simulink model "Encoder_polling"  (R2024b)
settings: Solver=FixedStepAuto  StartTime=0.0  StopTime=inf  FixedStep=0.001  RelTol=1e-3  EnableMultiTasking=on
libraries: stm32f4xxblockslib x5, stm32g4xxblockslib x3, simulink_extras x1
settings Model: STM32="{\"DigitalPortRead\":[{\"ID\":\"untitled:9\"},{\"ID\":\"untitled:10\"},{\"ID\":\"Encoder_Sim:129\"},{\"ID\":\"Encoder_Sim:130\"},{\"ID\":\"Encoder_Sim:134\"},{\"ID\":\"Encoder_Sim:135\"},{\"ID\":\"Encoder_Sim:299\"},{\"ID\":\"Encoder_polling:299\"},{\"ID\":\"Encoder_polling:130\"},{\"ID\":\"Encoder_polling:129\"},{\"ID\":\"Encoder_polling:135\"},{\"ID\":\"Encoder_polling:134\"}],\"EncoderBlockForG4\":[{\"ID\":\"untitled:13\"},{\"ID\":\"untitled:14\"},{\"ID\":\"untitled:15\"},{\"ID\":\"Encoder_Sim:13\"},{\"ID\":\"Encoder_Sim:14\"},{\"ID\":\"Encoder_Sim:15\"}]}"  Creator=chant  LastModifiedBy=pongn
settings OptimizationCC: BlockReduction=off  BooleanDataType=off  DefaultParameterBehavior=Inlined  EnhancedBackFolding=on  PassReuseOutputArgsAs=Individual arguments  ZeroExternalMemoryAtStartup=off  ZeroInternalMemoryAtStartup=off  MaxStackSize=512  OptimizeBlockOrder=speed  DifferentSizesBufferReuse=on  OptimizationCustomize=off  EfficientTunableParamExpr=on
settings DebuggingCC: SaveWithParameterizedLinksMsg=none  UnderspecifiedInitializationDetection=Classic  MergeDetectMultiDrivingBlocksExec=none  SignalResolutionControl=TryResolveAllWithWarning  ParameterTunabilityLossMsg=error
settings HardwareCC: ProdBitPerPointer=32  ProdBitPerSizeT=32  ProdBitPerPtrDiffT=32  ProdLargestAtomicInteger=Long  ProdLargestAtomicFloat=Double  ProdWordSize=32  ProdLongLongMode=on  ProdHWDeviceType=ARM Compatible->ARM Cortex-M
settings ModelReferenceCC: PropagateSignalLabelsOutOfModel=off
settings SFSimCC: MATLABDynamicMemAlloc=off
settings RTWCC: Description=Embedded Coder  SystemTargetFile=ert.tlc  HardwareBoard=STM32G4xx Based  TemplateMakefile=ert_default_tmf  Toolchain=GNU Tools for ARM Embedded Processors
settings CodeAppCC: ForceParamTrailComments=on  IgnoreCustomStorageClasses=off  OperatorAnnotations=on  SimulinkDataObjDesc=on  SFDataObjDesc=on  InsertBlockDesc=on
settings ERTTargetCC: TargetLangStandard=C99 (ISO)  CodeReplacementLibrary=ARM Cortex-M  SupportContinuousTime=on  ExtModeTransport=3  ExtModeStaticAlloc=on  ExtModeStaticAllocSize=2048  ExtModeMexFile=ext_xcp  ExtModeIntrfLevel=Level2 - Open

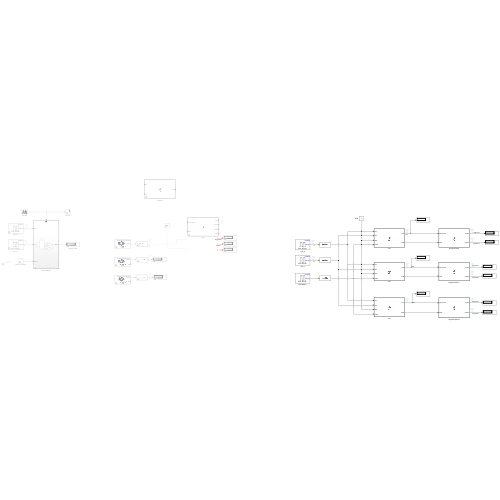
[thumbnail: Simulink's stored preview of the top-level diagram]
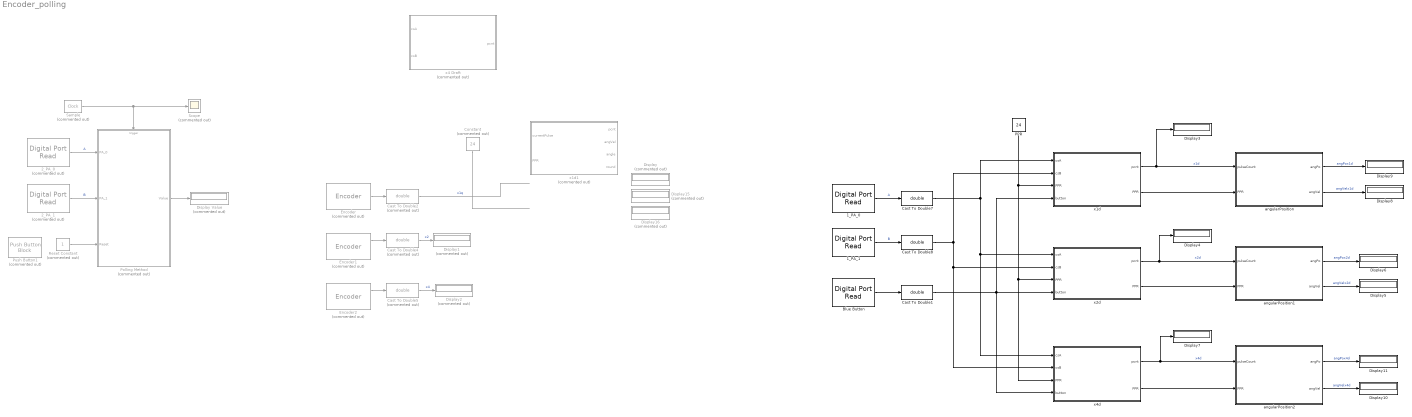
== system Encoder_polling ==
  1_PA_0 : stm32f4xxblockslib/Digital Port Read  PortName=GPIOA  PinNumber=[0]  ReadOperation=on  IOAsArray=on  SampleTime=-1  EnableSimPort=off  hoistedMaskSrc=ECSoC/ECSimCodegen/Digital Port Read
  1_PA_1 : stm32f4xxblockslib/Digital Port Read  PortName=GPIOA  PinNumber=[1]  ReadOperation=on  IOAsArray=on  SampleTime=-1  EnableSimPort=off  hoistedMaskSrc=ECSoC/ECSimCodegen/Digital Port Read
  2_PA_0 : stm32f4xxblockslib/Digital Port Read  Commented=on  PortName=GPIOA  PinNumber=[0]  ReadOperation=on  IOAsArray=on  SampleTime=-1  EnableSimPort=off  hoistedMaskSrc=ECSoC/ECSimCodegen/Digital Port Read
  2_PA_1 : stm32f4xxblockslib/Digital Port Read  Commented=on  PortName=GPIOA  PinNumber=[1]  ReadOperation=on  IOAsArray=on  SampleTime=-1  EnableSimPort=off  hoistedMaskSrc=ECSoC/ECSimCodegen/Digital Port Read
  Blue Button : stm32f4xxblockslib/Digital Port Read  PortName=GPIOC  PinNumber=[13]  ReadOperation=on  IOAsArray=on  SampleTime=-1  EnableSimPort=off  hoistedMaskSrc=ECSoC/ECSimCodegen/Digital Port Read
  Cast To Double1 : DataTypeConversion  OutDataTypeStr=double  SaturateOnIntegerOverflow=off  RndMeth=Floor
  Cast To Double2 : DataTypeConversion  Commented=on  OutDataTypeStr=double  SaturateOnIntegerOverflow=off  RndMeth=Floor
  Cast To Double4 : DataTypeConversion  Commented=on  OutDataTypeStr=double  SaturateOnIntegerOverflow=off  RndMeth=Floor
  Cast To Double5 : DataTypeConversion  Commented=on  OutDataTypeStr=double  SaturateOnIntegerOverflow=off  RndMeth=Floor
  Cast To Double7 : DataTypeConversion  OutDataTypeStr=double  SaturateOnIntegerOverflow=off  RndMeth=Floor
  Cast To Double8 : DataTypeConversion  OutDataTypeStr=double  SaturateOnIntegerOverflow=off  RndMeth=Floor
  Constant : Constant  Commented=on  Value=24
  Display{,1..2,15..16} (5 alike) : Display  Commented=on
  Display Value : Display  Commented=on
  Display{3..11} (9 alike) : Display
  Encoder : stm32g4xxblockslib/Encoder  Commented=on  TimerModule=TIM3  EnableResetInput=off  OutputCountAfterFirstIndex=off  OutputValidIndex=off  OutputDirection=off  OutputStatus=off  SampleTime=-1
  Encoder1 : stm32g4xxblockslib/Encoder  Commented=on  TimerModule=TIM4  EnableResetInput=off  OutputCountAfterFirstIndex=off  OutputValidIndex=off  OutputDirection=on  OutputStatus=off  SampleTime=-1
  Encoder2 : stm32g4xxblockslib/Encoder  Commented=on  TimerModule=TIM8  EnableResetInput=off  OutputCountAfterFirstIndex=off  OutputValidIndex=off  OutputDirection=on  OutputStatus=off  SampleTime=-1
  PPR : Constant  Value=24
  Polling Method : Subsystem  Commented=on
  Push Button1 : PushButtonBlock  Commented=on  OnValue=65521  OffValue=1.000000
  Reset Constant : Constant  Commented=on
  Sample : simulink_extras/Flip Flops/Clock  Commented=on  period=1
  Scope : Scope  Commented=on
  angularPosition : MATLAB Function  TreatAsAtomicUnit=on
  angularPosition1 : MATLAB Function  TreatAsAtomicUnit=on
  angularPosition2 : MATLAB Function  TreatAsAtomicUnit=on
  x1d : MATLAB Function  TreatAsAtomicUnit=on
  x1d1 : MATLAB Function  Commented=on  TreatAsAtomicUnit=on
  x2d : MATLAB Function  TreatAsAtomicUnit=on
  x4 Draft : MATLAB Function  Commented=on  TreatAsAtomicUnit=on
  x4d : MATLAB Function  TreatAsAtomicUnit=on
  wires:
  Sample/1 -> Polling Method/Trigger, Scope/1
  Polling Method/1(Value) -> Display Value/1
  Reset Constant/1 -> Polling Method/3(Reset)
  2_PA_1/1 -> Polling Method/2(PA_1)  "B"
  2_PA_0/1 -> Polling Method/1(PA_0)  "A"
  1_PA_0/1 -> Cast To Double7/1  "A"
  1_PA_1/1 -> Cast To Double8/1  "B"
  Cast To Double4/1 -> Display1/1  "x2"
  Cast To Double5/1 -> Display2/1  "x4"
  Encoder2/1 -> Cast To Double5/1
  Encoder1/1 -> Cast To Double4/1
  x1d/1(pcnt) -> Display3/1, angularPosition/1(pulseCount)  "x1d"
  Cast To Double7/1 -> x1d/1(csA), x4d/1(csA), x2d/1(csA)
  Cast To Double8/1 -> x4d/2(csB), x2d/2(csB), x1d/2(csB)
  angularPosition/2(angVel) -> Display8/1  "angVelx1d"
  angularPosition/1(angPo) -> Display9/1  "angPox1d"
  PPR/1 -> x4d/3("PPR "), x2d/3("PPR "), x1d/3("PPR ")
  x2d/1(pcnt) -> Display4/1, angularPosition1/1(pulseCount)  "x2d"
  angularPosition1/2(angVel) -> Display5/1  "angVelx2d"
  x4d/1(pcnt) -> Display7/1, angularPosition2/1(pulseCount)  "x4d"
  angularPosition2/2(angVel) -> Display10/1  "angVelx4d"
  Blue Button/1 -> Cast To Double1/1
  Cast To Double1/1 -> x4d/4(button), x1d/4(button), x2d/4(button)
  Encoder/1 -> Cast To Double2/1
  Cast To Double2/1 -> ?  "x1q"
  Constant/1 -> ?
  ? -> Display15/1  "angled"
  ? -> Display/1  "angVelx1q"
  ? -> Display16/1
  x1d/2(PPR) -> angularPosition/2(PPR)
  angularPosition1/1(angPo) -> Display6/1  "angPox2d"
  angularPosition2/1(angPo) -> Display11/1  "angPox4d"
  x4d/2(PPR) -> angularPosition2/2(PPR)
  x2d/2(PPR) -> angularPosition1/2(PPR)

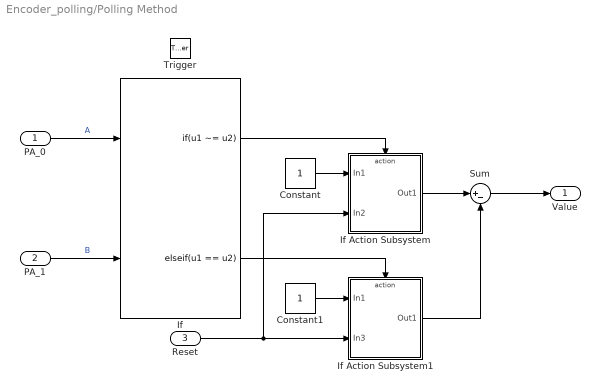
== system Encoder_polling/Polling Method ==
  PA_0 : Inport
  PA_1 : Inport  Port=2
  Reset : Inport  Port=3
  Trigger : TriggerPort  VariantControl=(inherit)  PortDimensions=1
  Constant : Constant
  Constant1 : Constant
  If : If  NumInputs=2  IfExpression=u1 ~= u2  ElseIfExpressions=u1 == u2  ShowElse=off
  If Action Subsystem : Subsystem  TreatAsAtomicUnit=on
  If Action Subsystem1 : Subsystem  TreatAsAtomicUnit=on
  Sum : Sum  Inputs=|+-
  Value : Outport
  wires:
  PA_1/1 -> If/2  "B"
  PA_0/1 -> If/1  "A"
  If/2 -> If Action Subsystem1/Action
  If/1 -> If Action Subsystem/Action
  Reset/1 -> If Action Subsystem1/2(In3), If Action Subsystem/2(In2)
  Constant/1 -> If Action Subsystem/1(In1)
  Constant1/1 -> If Action Subsystem1/1(In1)
  If Action Subsystem/1(Out1) -> Sum/1
  If Action Subsystem1/1(Out1) -> Sum/2
  Sum/1 -> Value/1

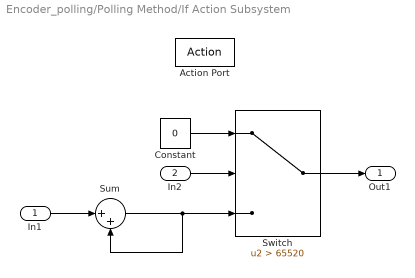
== system Encoder_polling/Polling Method/If Action Subsystem ==
  In1 : Inport
  In2 : Inport  Port=2
  Action Port : ActionPort  ActionPortLabel=if(u1 ~= u2)
  Constant : Constant  Value=0
  Sum : Sum  Inputs=|++
  Switch : Switch  Criteria=u2 > Threshold  Threshold=65520  SaturateOnIntegerOverflow=off  InputSameDT=off
  Out1 : Outport
  wires:
  In2/1 -> Switch/2
  Switch/1 -> Out1/1
  Constant/1 -> Switch/1
  Sum/1 -> Sum/2, Switch/3
  In1/1 -> Sum/1

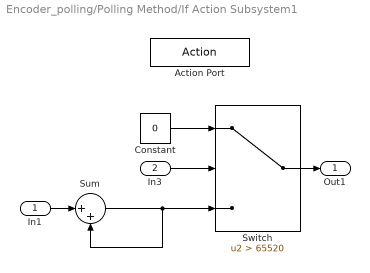
== system Encoder_polling/Polling Method/If Action Subsystem1 ==
  In1 : Inport
  In3 : Inport  Port=2
  Action Port : ActionPort  ActionPortLabel=elseif(u1 == u2)
  Constant : Constant  Value=0
  Sum : Sum  Inputs=|++
  Switch : Switch  Criteria=u2 > Threshold  Threshold=65520  SaturateOnIntegerOverflow=off  InputSameDT=off
  Out1 : Outport
  wires:
  In3/1 -> Switch/2
  Constant/1 -> Switch/1
  Sum/1 -> Sum/2, Switch/3
  In1/1 -> Sum/1
  Switch/1 -> Out1/1

== matlab function Encoder_polling/x1d1 ==
  data: currentPulse input; pcnt output; angVel output; angle output; PPR input; round output
function [pcnt, angVel, angle, round] = fcn(currentPulse, PPR)
    persistent psp lastTime;

    if isempty(psp)
        psp = 0;
        lastTime = tic;
    end

    ub = 65535-(mod(65535, PPR));
    lb = 0;

    if psp ~= currentPulse
        currentTime = toc(lastTime);
        angVel = (360 / PPR) / currentTime;
        lastTime = tic;
    else
        angVel = 0;
    end

    if pcnt_int < 24
        angle = pcnt_int * (360/PPR); % Angular position in degrees
        round = 0;
    else
        tempPulse = mod(pcnt_int, PPR);
        angle = mod(pcnt_int, PPR) * (360/PPR);
        round = (pcnt_int-tempPulse)/PPR;
    end

    pcnt = pcnt_int;
    psp = csA;
end

== matlab function Encoder_polling/x1d ==
  data: csA input; pcnt output; csB input; PPR input; button input; PPR output
function [pcnt, PPR] = fcn(csA, csB, PPR, button)
    persistent psA pcnt_int;

    if isempty(psA)
        psA = 0;
        pcnt_int = 0;
    end
    
    if button == 1
        pcnt_int = 0;
    end

    % Detect rising edge on csA
    if psA == 0 && csA == 1
        % Update pulse count based on direction (csB)
        if csB == 0  % Clockwise direction
            pcnt_int = pcnt_int + 1;
        elseif csB == 1  % Counterclockwise direction
            pcnt_int = pcnt_int - 1;
        end
    end
    
    pcnt = pcnt_int;
    psA = csA;
end

== matlab function Encoder_polling/angularPosition ==
  data: pulseCount input; angPo output; PPR input; angVel output
function [angPo, angVel] = fcn(pulseCount, PPR)
    % Define a persistent variable to retain previous pulse count across function calls
    persistent prev_pulseCount
    
    % Initialize persistent variable on the first function call
    if isempty(prev_pulseCount)
        prev_pulseCount = pulseCount;
        angVel = 0;       % Initialize angular velocity to zero
    else
        % Calculate the change in pulse count
        delta_pulseCount = pulseCount - prev_pulseCount;
        
        % Calculate angular velocity (radians per second)
        angVel = delta_pulseCount * ((2 * pi) / PPR) / 0.01;
        
        % Update previous pulse count for the next calculation
        prev_pulseCount = pulseCount;
    end

    % Calculate angular position (in radians)
    angPo = pulseCount * ((2 * pi) / PPR);
end

== matlab function Encoder_polling/x4 Draft ==
  data: csA input; pcnt output; csB input
function pcnt = fcn(csA, csB) % มีอินพุตเป็น csA และ csB โดยมันีเอาพุตเป็น pcnt

ub = int32(65520); % ขอบบน (65535-mod(65535))
lb = int32(0);     % ขอบล่าง (0)

persistent psA psB;   % Previous State A and B
persistent pcnt_int;  % Pulse Count Internal

if isempty(psA) % เช็คว่า psA ว่างหรือเปล่า ถ้าว่างให้เป็นจริง
    psA = int32(0); % ให้ psA เป็น 0
end

if isempty(psB) % เช็คว่า psB ว่างหรือเปล่า ถ้าว่างให้เป็นจริง
    psB = int32(0); % ให้ psB เป็น 0
end

if isempty(pcnt_int) % เช็คว่า pcnt_int ว่างหรือเปล่า ถ้าว่างให้เป็นจริง
    pcnt_int = int32(-1); % Offset
end

csA = int32(csA(1)); % Current State A
csB = int32(csB(1)); % Current State B

if psA ~= csA || psB ~= csB  % เกิดการเปลี่ยนแปลงของ state A และ B
    if (psA == 0 && csA == 1 && csB == 0) || ...  % Rising A, B = 0
       (psB == 0 && csB == 1 && csA == 1) || ...  % Rising B, A = 1
       (psA == 1 && csA == 0 && csB == 1) || ...  % Falling A, B = 1
       (psB == 1 && csB == 0 && csA == 0)         % Falling B, A = 0
        pcnt_int = pcnt_int + int32(1);  % ตามเข็มนาฬิกา
    else
        pcnt_int = pcnt_int - int32(1);  % ทวนเข็มนาฬิกา
    end

    % การ Overflow และ Limited Boundary
    if pcnt_int < lb
        pcnt_int = ub;
    elseif pcnt_int > ub
        pcnt_int = lb;
    end
end

pcnt = pcnt_int;  % เอาพุตเป็นค่า pcnt_int

psA = csA; % อัพเดท state A
psB = csB; % อัพเดท state B
end

== matlab function Encoder_polling/x2d ==
  data: csA input; pcnt output; csB input; PPR input; PPR output; button input
function [pcnt, PPR] = fcn(csA, csB, PPR, button)
    persistent psA pcnt_int;
    
    if isempty(psA)
        psA = 0;
        pcnt_int = 0;
    end

    if button == 1
        pcnt_int = 0;
    end

    % Detect rising edge on csA
    if psA ~= csA
        if csA == 1  % Rising edge (0 -> 1)
            if csB == 0  % ตามเข็มนาฬิกา
                pcnt_int = pcnt_int + 1;  % เพิ่ม 1
            else  % ทวนเข็มนาฬิกา
                pcnt_int = pcnt_int - 1;  % ลด 1
            end
        elseif csA == 0  % Falling edge (1 -> 0)
            if csB == 1  % ตามเข็มนาฬิกา
                pcnt_int = pcnt_int + 1;  % เพิ่ม 1
            else  % ทวนเข็มนาฬิกา
                pcnt_int = pcnt_int - 1;  % ลด 1
            end
        end
    end
    pcnt = pcnt_int;
    psA = csA;
end

== matlab function Encoder_polling/x4d ==
  data: csA input; pcnt output; csB input; PPR input; PPR output; button input
function [pcnt, PPR] = fcn(csA, csB, PPR, button)
    persistent psA psB pcnt_int;

    if isempty(psA)
        psA = 0;
        psB = 0;
        pcnt_int = 0;
    end

    if button == 1
        pcnt_int = 0;
    end

    % Detect rising edge on csA
    if psA ~= csA || psB ~= csB
        if psA ~= csA || psB ~= csB  % เกิดการเปลี่ยนแปลงของ state A และ B
            if (psA == 0 && csA == 1 && csB == 0) || ...  % Rising A, B = 0
                (psB == 0 && csB == 1 && csA == 1) || ...  % Rising B, A = 1
                (psA == 1 && csA == 0 && csB == 1) || ...  % Falling A, B = 1
                (psB == 1 && csB == 0 && csA == 0)         % Falling B, A = 0
                    pcnt_int = pcnt_int + 1;  % ตามเข็มนาฬิกา
            else
                    pcnt_int = pcnt_int - 1;  % ทวนเข็มนาฬิกา
            end
        end
    end
    pcnt = pcnt_int;
    psA = csA;
    psB = csB;
end

== matlab function Encoder_polling/angularPosition1 ==
  data: pulseCount input; angPo output; PPR input; angVel output
function [angPo, angVel] = fcn(pulseCount, PPR)
    % Define a persistent variable to retain previous pulse count across function calls
    persistent prev_pulseCount
    
    % Initialize persistent variable on the first function call
    if isempty(prev_pulseCount)
        prev_pulseCount = pulseCount;
        angVel = 0;       % Initialize angular velocity to zero
    else
        % Calculate the change in pulse count
        delta_pulseCount = pulseCount - prev_pulseCount;
        
        % Calculate angular velocity (radians per second)
        angVel = delta_pulseCount * ((2 * pi) / PPR) / 0.01;
        
        % Update previous pulse count for the next calculation
        prev_pulseCount = pulseCount;
    end

    % Calculate angular position (in radians)
    angPo = pulseCount * ((2 * pi) / PPR);
end

== matlab function Encoder_polling/angularPosition2 ==
  data: pulseCount input; angPo output; PPR input; angVel output
function [angPo, angVel] = fcn(pulseCount, PPR)
    % Define a persistent variable to retain previous pulse count across function calls
    persistent prev_pulseCount
    
    % Initialize persistent variable on the first function call
    if isempty(prev_pulseCount)
        prev_pulseCount = pulseCount;
        angVel = 0;       % Initialize angular velocity to zero
    else
        % Calculate the change in pulse count
        delta_pulseCount = pulseCount - prev_pulseCount;
        
        % Calculate angular velocity (radians per second)
        angVel = delta_pulseCount * ((2 * pi) / PPR) / 0.01;
        
        % Update previous pulse count for the next calculation
        prev_pulseCount = pulseCount;
    end

    % Calculate angular position (in radians)
    angPo = pulseCount * ((2 * pi) / PPR);
end
